simulink model "sim_Planar6DoF"  (R2017b)
settings: Solver=FixedStepAuto  StartTime=0.0  StopTime=t_end  FixedStep=Ts  RelTol=1e-3
PreLoadFcn:
  | init_sim_Planar6DoF
StopFcn:
  | runVisualization
undefined symbols (not defined in the file): B_theta, D_JointImp, D_theta, DiscIntNeverNeededParam, dq0, dq_init, K, K_JointImp, K_theta, M_des, Nb, Omega, q0, q0_offset, ROBOT, Ts
libraries: simulink x6
(part 1 of 2)
settings Model: Creator=wu_xw  LastModifiedBy=diet_ae

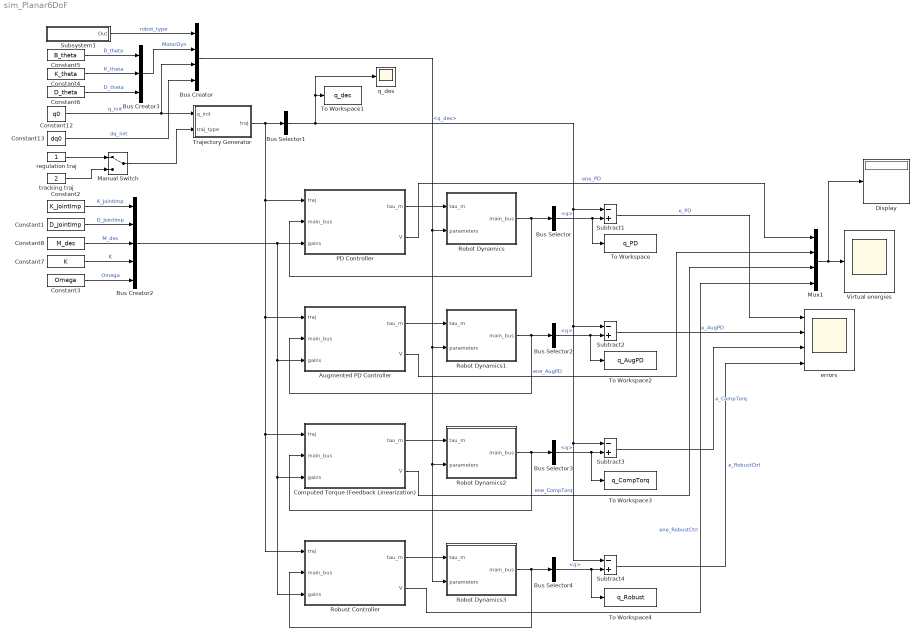
== system sim_Planar6DoF ==
  Augmented PD Controller : Subsystem
  Bus Creator : BusCreator  Inputs=4
  Bus Creator2 : BusCreator  Inputs=5
  Bus Creator3 : BusCreator  Inputs=3
  Bus Selector{,2..4} (4 alike) : BusSelector  OutputSignals=States.q
  Bus Selector1 : BusSelector  OutputSignals=q_des
  Computed Torque (Feedback Linearization) : Subsystem
  Constant1 : Constant  Value=D_JointImp  SampleTime=-1
  Constant12 : Constant  Value=q0  SampleTime=-1
  Constant13 : Constant  Value=dq0  SampleTime=-1
  Constant2 : Constant  Value=K_JointImp  SampleTime=-1
  Constant3 : Constant  Value=Omega  SampleTime=-1
  Constant4 : Constant  Value=K_theta
  Constant5 : Constant  Value=B_theta
  Constant6 : Constant  Value=D_theta
  Constant7 : Constant  Value=K  SampleTime=-1
  Constant8 : Constant  Value=M_des  SampleTime=-1
  Display : Display
  Manual Switch : ManualSwitch
  Mux1 : Mux
  PD Controller : Subsystem
  Robot Dynamics : Subsystem
      settings: MinAlgLoopOccurrences=on
      mask Display: image('Planar6DoF.png');
  Robot Dynamics1 : Subsystem
      settings: MinAlgLoopOccurrences=on
      mask Display: image('Planar6DoF.png');
  Robot Dynamics2 : Subsystem
      settings: MinAlgLoopOccurrences=on
      mask Display: image('Planar6DoF.png');
  Robot Dynamics3 : Subsystem
      settings: MinAlgLoopOccurrences=on
      mask Display: image('Planar6DoF.png');
  Robust Controller : Subsystem
  Subsystem1 : Subsystem  mask{select=1. Rigid Robot}
      mask prompts: select "Parameters are specified in"
      mask init:
      | mytab={'1. Rigid Robot',...
      |        '2. Flexible Joint Robot'};
      mask TypeOptions select: 1. Rigid Robot | 2. Flexible Joint Robot
      mask Display: disp(mytab{select});
  Subtract{1..4} (4 alike) : Sum  Inputs=-+
  To Workspace : ToWorkspace  VariableName=q_PD  SampleTime=-1
      settings: Save2DSignal=2-D array (concatenate along first dimension)
  To Workspace1 : ToWorkspace  VariableName=q_des  SampleTime=-1
      settings: Save2DSignal=2-D array (concatenate along first dimension)
  To Workspace2 : ToWorkspace  VariableName=q_AugPD  SampleTime=-1
      settings: Save2DSignal=2-D array (concatenate along first dimension)
  To Workspace3 : ToWorkspace  VariableName=q_CompTorq  SampleTime=-1
      settings: Save2DSignal=2-D array (concatenate along first dimension)
  To Workspace4 : ToWorkspace  VariableName=q_Robust  SampleTime=-1
      settings: Save2DSignal=2-D array (concatenate along first dimension)
  Trajectory Generator : Subsystem
  Virtual energies : Scope
  errors : Scope  NumInputPorts=4
  q_des : Scope
  regulation traj : Constant
  tracking traj : Constant  Value=2
  wires:
  Robot Dynamics/1(main_bus) -> Bus Selector/1, PD Controller/2(main_bus)
  PD Controller/1(tau_m) -> Robot Dynamics/1(tau_m)
  Bus Selector/1 -> Subtract1/2, To Workspace/1  "<q>"
  Constant6/1 -> Bus Creator3/3  "D_theta"
  Constant5/1 -> Bus Creator3/1  "B_theta"
  Bus Creator3/1 -> Bus Creator/2  "MotorDyn"
  Constant4/1 -> Bus Creator3/2  "K_theta"
  Constant13/1 -> Bus Creator/4  "dq_init"
  Constant12/1 -> Trajectory Generator/1(q_init), Bus Creator/3  "q_init"
  Subsystem1/1(Out) -> Bus Creator/1  "robot_type"
  Constant1/1 -> Bus Creator2/2  "D_JointImp"
  Constant2/1 -> Bus Creator2/1  "K_JointImp"
  Augmented PD Controller/1(tau_m) -> Robot Dynamics1/1(tau_m)
  Robot Dynamics2/1(main_bus) -> Bus Selector3/1, Computed Torque (Feedback Linearization)/2(main_bus)
  Computed Torque (Feedback Linearization)/1(tau_m) -> Robot Dynamics2/1(tau_m)
  Bus Selector2/1 -> To Workspace2/1, Subtract2/2  "<q>"
  Robot Dynamics1/1(main_bus) -> Augmented PD Controller/2(main_bus), Bus Selector2/1
  Bus Selector3/1 -> To Workspace3/1, Subtract3/2  "<q>"
  regulation traj/1 -> Manual Switch/1
  tracking traj/1 -> Manual Switch/2
  Manual Switch/1 -> Trajectory Generator/2(traj_type)
  Subtract1/1 -> errors/1  "e_PD"
  Subtract2/1 -> errors/2  "e_AugPD"
  Subtract3/1 -> errors/3  "e_CompTorq"
  Subtract4/1 -> errors/4  "e_RobustCtrl"
  Bus Selector1/1 -> q_des/1, To Workspace1/1, Subtract4/1, Subtract3/1, Subtract2/1, Subtract1/1  "<q_des>"
  Bus Selector4/1 -> To Workspace4/1, Subtract4/2  "<q>"
  Bus Creator/1 -> Robot Dynamics/2(parameters), Robot Dynamics3/2(parameters), Robot Dynamics2/2(parameters), Robot Dynamics1/2(parameters)
  Trajectory Generator/1(traj) -> Robust Controller/1(traj), Computed Torque (Feedback Linearization)/1(traj), Augmented PD Controller/1(traj), PD Controller/1(traj), Bus Selector1/1
  Robust Controller/1(tau_m) -> Robot Dynamics3/1(tau_m)
  Robot Dynamics3/1(main_bus) -> Robust Controller/2(main_bus), Bus Selector4/1
  Bus Creator2/1 -> Augmented PD Controller/3(gains), Robust Controller/3(gains), Computed Torque (Feedback Linearization)/3(gains), PD Controller/3(gains)
  Constant7/1 -> Bus Creator2/4  "K"
  Constant3/1 -> Bus Creator2/5  "Omega"
  Constant8/1 -> Bus Creator2/3  "M_des"
  PD Controller/2(V) -> Mux1/1  "ene_PD"
  Augmented PD Controller/2(V) -> Mux1/2  "ene_AugPD"
  Computed Torque (Feedback Linearization)/2(V) -> Mux1/3  "ene_CompTorq"
  Robust Controller/2(V) -> Mux1/4  "ene_RobustCtrl"
  Mux1/1 -> Display/1, Virtual energies/1

== system sim_Planar6DoF/Augmented PD Controller ==
  traj : Inport
  main_bus : Inport  Port=2
  gains : Inport  Port=3
  Bus Selector : BusSelector  OutputSignals=Dyn.M,Dyn.CC,Dyn.g,States.q,States.dq
  Bus Selector1 : BusSelector  OutputSignals=K_JointImp,D_JointImp
  Bus Selector2 : BusSelector  OutputSignals=q_des,dq_des,ddq_des
  Product{1..4} (4 alike) : Product  Multiplication=Matrix(*)  RndMeth=Zero
  Storage Function : Subsystem  TreatAsAtomicUnit=on
      settings: RTWFcnNameOpts=Use subsystem name  RTWFileNameOpts=Use function name
  Subtract : Sum  Inputs=+-
  Subtract1 : Sum  Inputs=--
  Subtract2 : Sum  Inputs=++++
  Subtract3 : Sum  Inputs=+-
  tau_m : Outport
  V : Outport  Port=2
  wires:
  Product4/1 -> Subtract2/2
  Bus Selector/2 -> Product4/1  "<CC>"
  Bus Selector/1 -> Storage Function/1(M), Product3/1  "<M>"
  Bus Selector2/3 -> Product3/2  "<ddq_des>"
  Subtract3/1 -> Product2/2, Storage Function/4(de)
  Bus Selector2/2 -> Subtract3/2, Product4/2  "<dq_des>"
  Bus Selector/5 -> Subtract3/1  "<dq>"
  Bus Selector2/1 -> Subtract/2  "<q_des>"
  Bus Selector/3 -> Subtract2/3  "<g>"
  Product3/1 -> Subtract2/1
  Product2/1 -> Subtract1/2
  Product1/1 -> Subtract1/1
  Bus Selector1/2 -> Product2/1  "<D_JointImp>"
  Bus Selector1/1 -> Storage Function/2(K), Product1/1  "<K_JointImp>"
  Subtract/1 -> Storage Function/3(e), Product1/2
  traj/1 -> Bus Selector2/1
  Bus Selector/4 -> Subtract/1  "<q>"
  gains/1 -> Bus Selector1/1
  main_bus/1 -> Bus Selector/1
  Subtract2/1 -> tau_m/1
  Subtract1/1 -> Subtract2/4
  Storage Function/1(V) -> V/1

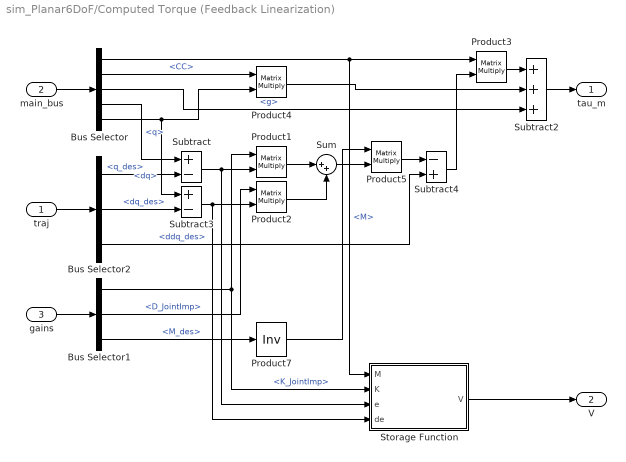
== system sim_Planar6DoF/Computed Torque (Feedback Linearization) ==
  traj : Inport
  main_bus : Inport  Port=2
  gains : Inport  Port=3
  Bus Selector : BusSelector  OutputSignals=Dyn.M,Dyn.CC,Dyn.g,States.q,States.dq
  Bus Selector1 : BusSelector  OutputSignals=K_JointImp,D_JointImp,M_des
  Bus Selector2 : BusSelector  OutputSignals=q_des,dq_des,ddq_des
  Product{1..5} (5 alike) : Product  Multiplication=Matrix(*)  RndMeth=Zero
  Product7 : Product  Inputs=/  Multiplication=Matrix(*)  RndMeth=Zero
  Storage Function : Subsystem  TreatAsAtomicUnit=on
      settings: RTWFcnNameOpts=Use subsystem name  RTWFileNameOpts=Use function name
  Subtract : Sum  Inputs=+-
  Subtract2 : Sum  Inputs=+++
  Subtract3 : Sum  Inputs=+-
  Subtract4 : Sum  Inputs=-+
  Sum : Sum  Inputs=|++
  tau_m : Outport
  V : Outport  Port=2
  wires:
  main_bus/1 -> Bus Selector/1
  Subtract2/1 -> tau_m/1
  gains/1 -> Bus Selector1/1
  Bus Selector/4 -> Subtract/1  "<q>"
  traj/1 -> Bus Selector2/1
  Subtract/1 -> Storage Function/3(e), Product1/2
  Bus Selector1/1 -> Storage Function/2(K), Product1/1  "<K_JointImp>"
  Bus Selector1/2 -> Product2/1  "<D_JointImp>"
  Product1/1 -> Sum/1
  Product2/1 -> Sum/2
  Product3/1 -> Subtract2/1
  Bus Selector/3 -> Subtract2/3  "<g>"
  Bus Selector2/1 -> Subtract/2  "<q_des>"
  Bus Selector/5 -> Product4/2, Subtract3/1  "<dq>"
  Bus Selector2/2 -> Subtract3/2  "<dq_des>"
  Subtract3/1 -> Storage Function/4(de), Product2/2
  Bus Selector2/3 -> Subtract4/2  "<ddq_des>"
  Subtract4/1 -> Product3/2
  Bus Selector/1 -> Storage Function/1(M), Product3/1  "<M>"
  Bus Selector/2 -> Product4/1  "<CC>"
  Product4/1 -> Subtract2/2
  Bus Selector1/3 -> Product7/1  "<M_des>"
  Sum/1 -> Product5/2
  Product5/1 -> Subtract4/1
  Product7/1 -> Product5/1
  Storage Function/1(V) -> V/1

== system sim_Planar6DoF/PD Controller ==
  traj : Inport
  main_bus : Inport  Port=2
  gains : Inport  Port=3
  Bus Selector : BusSelector  OutputSignals=Dyn.g,States.q,States.dq,Dyn.M
  Bus Selector1 : BusSelector  OutputSignals=K_JointImp,D_JointImp
  Bus Selector2 : BusSelector  OutputSignals=q_des,dq_des
  Gain : Gain  Gain=-1
  Product1 : Product  Multiplication=Matrix(*)  RndMeth=Zero
  Product2 : Product  Multiplication=Matrix(*)  RndMeth=Zero
  Storage Function : Subsystem  TreatAsAtomicUnit=on
      settings: RTWFcnNameOpts=Use subsystem name  RTWFileNameOpts=Use function name
  Subtract : Sum  Inputs=+-
  Subtract1 : Sum
  Subtract2 : Sum
  Subtract3 : Sum  Inputs=+-
  tau_m : Outport
  V : Outport  Port=2
  wires:
  main_bus/1 -> Bus Selector/1
  Bus Selector/3 -> Subtract3/1, Product2/2  "<dq>"
  Subtract2/1 -> tau_m/1
  gains/1 -> Bus Selector1/1
  Bus Selector/2 -> Subtract/1  "<q>"
  traj/1 -> Bus Selector2/1
  Subtract/1 -> Storage Function/3(e), Product1/2
  Bus Selector1/1 -> Storage Function/2(K), Product1/1  "<K_JointImp>"
  Bus Selector1/2 -> Product2/1  "<D_JointImp>"
  Product1/1 -> Subtract1/1
  Product2/1 -> Subtract1/2
  Subtract1/1 -> Gain/1
  Gain/1 -> Subtract2/2
  Bus Selector/1 -> Subtract2/1  "<g>"
  Bus Selector2/1 -> Subtract/2  "<q_des>"
  Bus Selector/4 -> Storage Function/1(M)  "<M>"
  Subtract3/1 -> Storage Function/4(de)
  Bus Selector2/2 -> Subtract3/2  "<dq_des>"
  Storage Function/1(V) -> V/1

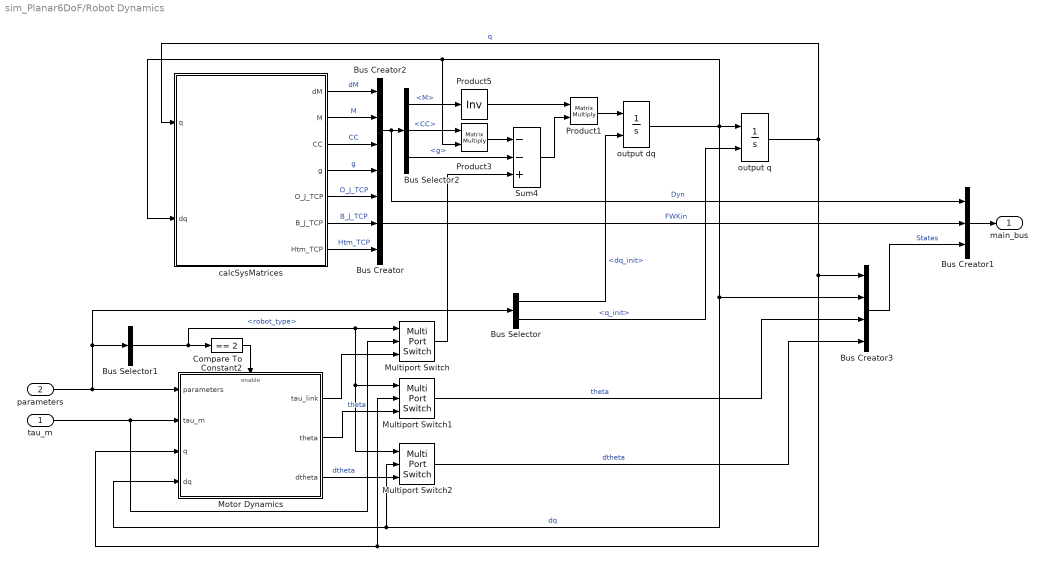
== system sim_Planar6DoF/Robot Dynamics ==
  tau_m : Inport
  parameters : Inport  Port=2
  Bus Creator : BusCreator  Inputs=3
  Bus Creator1 : BusCreator  Inputs=3
  Bus Creator2 : BusCreator  Inputs=4
  Bus Creator3 : BusCreator  Inputs=4
  Bus Selector : BusSelector  OutputSignals=dq_init,q_init
  Bus Selector1 : BusSelector  OutputSignals=robot_type
  Bus Selector2 : BusSelector  OutputSignals=M,CC,g
  Compare To Constant2 : simulink/Logic and Bit Operations/Compare To Constant  relop===  const=2  OutDataTypeStr=boolean
  Motor Dynamics : Subsystem  TreatAsAtomicUnit=on
  Multiport Switch : MultiPortSwitch  Inputs=2
  Multiport Switch1 : MultiPortSwitch  Inputs=2
  Multiport Switch2 : MultiPortSwitch  Inputs=2
  Product1 : Product  Multiplication=Matrix(*)  RndMeth=Zero
  Product3 : Product  Multiplication=Matrix(*)  RndMeth=Zero
  Product5 : Product  Inputs=/  Multiplication=Matrix(*)  RndMeth=Zero
  Sum4 : Sum  Inputs=--+
  calcSysMatrices : MATLAB Function  TreatAsAtomicUnit=on  mask{ROBOT=ROBOT}
      mask prompts: ROBOT "Robot Model"
      mask help:
      | Calculates inertia and coriolis compensation matrices
      |
      | A MATLAB structure ROBOT with the fields:
      |
      | g0 - matrix stacking vertically the homogeneous transformation matrices from parent to link in the zero-configuration
      | csi - vector stacking vertically the 6-by-1 relative body jacobian (twist) in link frame
      | Mass - block diagonal matrix, where each block is the 6-by-6 inertia matrix of the link in link frame
      |
      | must be initialized in workspace.
  output dq : Integrator  InitialConditionSource=external  InitialCondition=[zeros(Nb,1); dq_init]
  output q : Integrator  InitialConditionSource=external  InitialCondition=[zeros(Nb,1); dq_init]
  main_bus : Outport
  wires:
  Sum4/1 -> Product1/2
  parameters/1 -> Bus Selector/1, Bus Selector1/1, Motor Dynamics/1(parameters)
  Bus Selector/1 -> output dq/2  "<dq_init>"
  Product1/1 -> output dq/1
  Bus Creator1/1 -> main_bus/1
  Product3/1 -> Sum4/1
  Bus Selector/2 -> output q/2  "<q_init>"
  calcSysMatrices/2(M) -> Bus Creator2/2  "M"
  Product5/1 -> Product1/1
  calcSysMatrices/3(CC) -> Bus Creator2/3  "CC"
  output dq/1 -> output q/1, calcSysMatrices/2(dq), Product3/2, Bus Creator3/2, Multiport Switch2/2, Motor Dynamics/4(dq)  "dq"
  calcSysMatrices/4(g) -> Bus Creator2/4  "g"
  calcSysMatrices/5(O_J_TCP) -> Bus Creator/1  "O_J_TCP"
  calcSysMatrices/6(B_J_TCP) -> Bus Creator/2  "B_J_TCP"
  calcSysMatrices/7(Htm_TCP) -> Bus Creator/3  "Htm_TCP"
  Bus Creator/1 -> Bus Creator1/2  "FWKin"
  Bus Selector1/1 -> Multiport Switch2/1, Multiport Switch1/1, Multiport Switch/1, Compare To Constant2/1  "<robot_type>"
  Compare To Constant2/1 -> Motor Dynamics/Enable
  tau_m/1 -> Multiport Switch/2, Motor Dynamics/2(tau_m)
  Motor Dynamics/1(tau_link) -> Multiport Switch/3
  Multiport Switch1/1 -> Bus Creator3/3  "theta"
  Multiport Switch2/1 -> Bus Creator3/4  "dtheta"
  Multiport Switch/1 -> Sum4/3
  Motor Dynamics/2(theta) -> Multiport Switch1/3  "theta"
  Motor Dynamics/3(dtheta) -> Multiport Switch2/3  "dtheta"
  Bus Creator3/1 -> Bus Creator1/3  "States"
  calcSysMatrices/1(dM) -> Bus Creator2/1  "dM"
  Bus Creator2/1 -> Bus Creator1/1, Bus Selector2/1  "Dyn"
  Bus Selector2/1 -> Product5/1  "<M>"
  Bus Selector2/2 -> Product3/1  "<CC>"
  Bus Selector2/3 -> Sum4/2  "<g>"
  output q/1 -> calcSysMatrices/1(q), Bus Creator3/1, Multiport Switch1/2, Motor Dynamics/3(q)  "q"

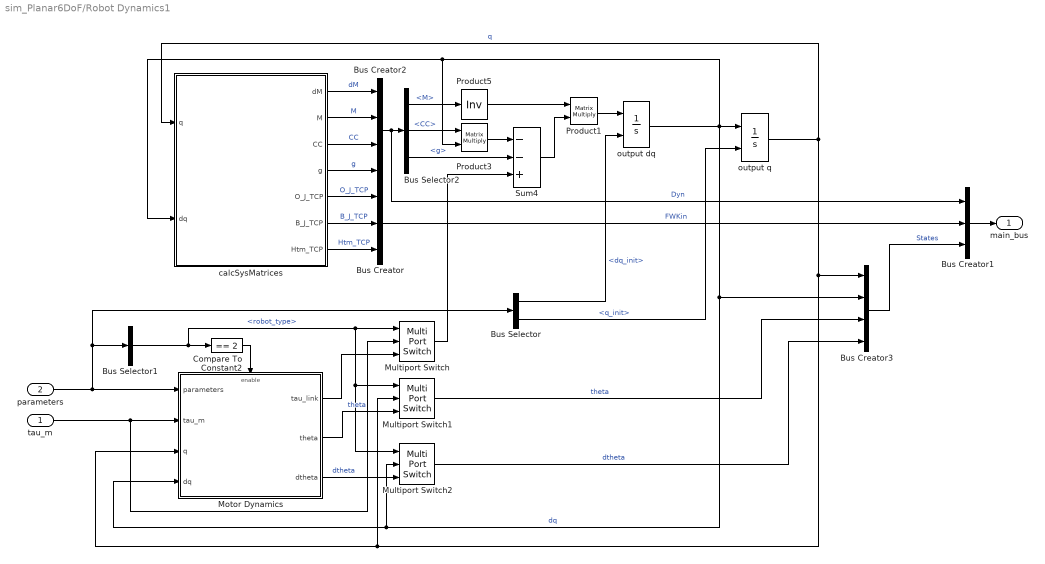
== system sim_Planar6DoF/Robot Dynamics1 ==
  tau_m : Inport
  parameters : Inport  Port=2
  Bus Creator : BusCreator  Inputs=3
  Bus Creator1 : BusCreator  Inputs=3
  Bus Creator2 : BusCreator  Inputs=4
  Bus Creator3 : BusCreator  Inputs=4
  Bus Selector : BusSelector  OutputSignals=dq_init,q_init
  Bus Selector1 : BusSelector  OutputSignals=robot_type
  Bus Selector2 : BusSelector  OutputSignals=M,CC,g
  Compare To Constant2 : simulink/Logic and Bit Operations/Compare To Constant  relop===  const=2  OutDataTypeStr=boolean
  Motor Dynamics : Subsystem  TreatAsAtomicUnit=on
  Multiport Switch : MultiPortSwitch  Inputs=2
  Multiport Switch1 : MultiPortSwitch  Inputs=2
  Multiport Switch2 : MultiPortSwitch  Inputs=2
  Product1 : Product  Multiplication=Matrix(*)  RndMeth=Zero
  Product3 : Product  Multiplication=Matrix(*)  RndMeth=Zero
  Product5 : Product  Inputs=/  Multiplication=Matrix(*)  RndMeth=Zero
  Sum4 : Sum  Inputs=--+
  calcSysMatrices : MATLAB Function  TreatAsAtomicUnit=on  mask{ROBOT=ROBOT}
      mask prompts: ROBOT "Robot Model"
      mask help:
      | Calculates inertia and coriolis compensation matrices
      |
      | A MATLAB structure ROBOT with the fields:
      |
      | g0 - matrix stacking vertically the homogeneous transformation matrices from parent to link in the zero-configuration
      | csi - vector stacking vertically the 6-by-1 relative body jacobian (twist) in link frame
      | Mass - block diagonal matrix, where each block is the 6-by-6 inertia matrix of the link in link frame
      |
      | must be initialized in workspace.
  output dq : Integrator  InitialConditionSource=external  InitialCondition=[zeros(Nb,1); dq_init]
  output q : Integrator  InitialConditionSource=external  InitialCondition=[zeros(Nb,1); dq_init]
  main_bus : Outport
  wires:
  output q/1 -> Motor Dynamics/3(q), Multiport Switch1/2, Bus Creator3/1, calcSysMatrices/1(q)  "q"
  Bus Selector2/3 -> Sum4/2  "<g>"
  Bus Selector2/2 -> Product3/1  "<CC>"
  Bus Selector2/1 -> Product5/1  "<M>"
  Bus Creator2/1 -> Bus Selector2/1, Bus Creator1/1  "Dyn"
  calcSysMatrices/1(dM) -> Bus Creator2/1  "dM"
  Bus Creator3/1 -> Bus Creator1/3  "States"
  Motor Dynamics/3(dtheta) -> Multiport Switch2/3  "dtheta"
  Motor Dynamics/2(theta) -> Multiport Switch1/3  "theta"
  Multiport Switch/1 -> Sum4/3
  Multiport Switch2/1 -> Bus Creator3/4  "dtheta"
  Multiport Switch1/1 -> Bus Creator3/3  "theta"
  Motor Dynamics/1(tau_link) -> Multiport Switch/3
  tau_m/1 -> Motor Dynamics/2(tau_m), Multiport Switch/2
  Compare To Constant2/1 -> Motor Dynamics/Enable
  Bus Selector1/1 -> Compare To Constant2/1, Multiport Switch/1, Multiport Switch1/1, Multiport Switch2/1  "<robot_type>"
  Bus Creator/1 -> Bus Creator1/2  "FWKin"
  calcSysMatrices/7(Htm_TCP) -> Bus Creator/3  "Htm_TCP"
  calcSysMatrices/6(B_J_TCP) -> Bus Creator/2  "B_J_TCP"
  calcSysMatrices/5(O_J_TCP) -> Bus Creator/1  "O_J_TCP"
  calcSysMatrices/4(g) -> Bus Creator2/4  "g"
  output dq/1 -> Motor Dynamics/4(dq), Multiport Switch2/2, Bus Creator3/2, Product3/2, calcSysMatrices/2(dq), output q/1  "dq"
  calcSysMatrices/3(CC) -> Bus Creator2/3  "CC"
  Product5/1 -> Product1/1
  calcSysMatrices/2(M) -> Bus Creator2/2  "M"
  Bus Selector/2 -> output q/2  "<q_init>"
  Product3/1 -> Sum4/1
  Bus Creator1/1 -> main_bus/1
  Product1/1 -> output dq/1
  Bus Selector/1 -> output dq/2  "<dq_init>"
  parameters/1 -> Motor Dynamics/1(parameters), Bus Selector1/1, Bus Selector/1
  Sum4/1 -> Product1/2

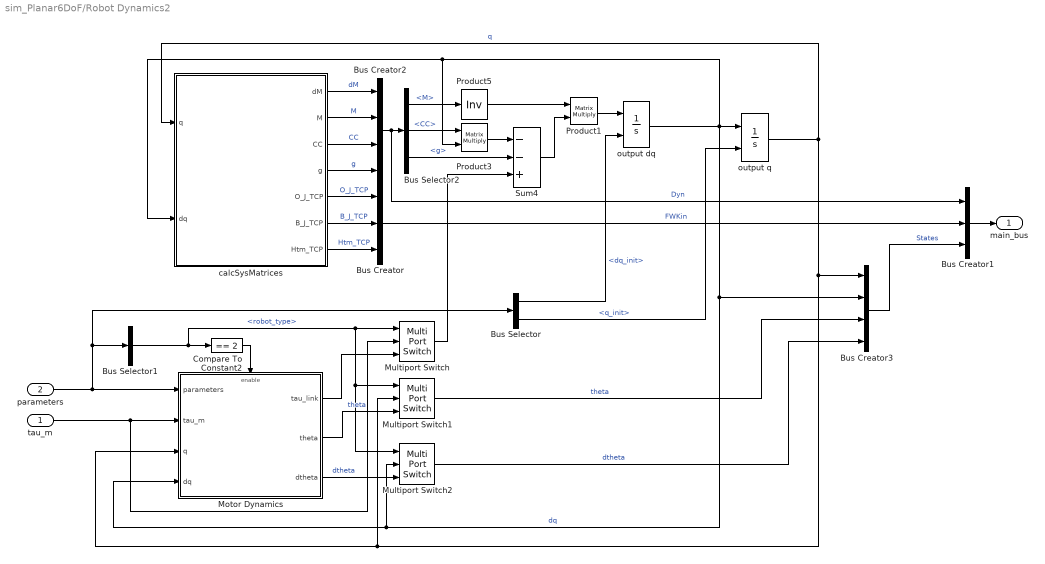
== system sim_Planar6DoF/Robot Dynamics2 ==
  tau_m : Inport
  parameters : Inport  Port=2
  Bus Creator : BusCreator  Inputs=3
  Bus Creator1 : BusCreator  Inputs=3
  Bus Creator2 : BusCreator  Inputs=4
  Bus Creator3 : BusCreator  Inputs=4
  Bus Selector : BusSelector  OutputSignals=dq_init,q_init
  Bus Selector1 : BusSelector  OutputSignals=robot_type
  Bus Selector2 : BusSelector  OutputSignals=M,CC,g
  Compare To Constant2 : simulink/Logic and Bit Operations/Compare To Constant  relop===  const=2  OutDataTypeStr=boolean
  Motor Dynamics : Subsystem  TreatAsAtomicUnit=on
  Multiport Switch : MultiPortSwitch  Inputs=2
  Multiport Switch1 : MultiPortSwitch  Inputs=2
  Multiport Switch2 : MultiPortSwitch  Inputs=2
  Product1 : Product  Multiplication=Matrix(*)  RndMeth=Zero
  Product3 : Product  Multiplication=Matrix(*)  RndMeth=Zero
  Product5 : Product  Inputs=/  Multiplication=Matrix(*)  RndMeth=Zero
  Sum4 : Sum  Inputs=--+
  calcSysMatrices : MATLAB Function  TreatAsAtomicUnit=on  mask{ROBOT=ROBOT}
      mask prompts: ROBOT "Robot Model"
      mask help:
      | Calculates inertia and coriolis compensation matrices
      |
      | A MATLAB structure ROBOT with the fields:
      |
      | g0 - matrix stacking vertically the homogeneous transformation matrices from parent to link in the zero-configuration
      | csi - vector stacking vertically the 6-by-1 relative body jacobian (twist) in link frame
      | Mass - block diagonal matrix, where each block is the 6-by-6 inertia matrix of the link in link frame
      |
      | must be initialized in workspace.
  output dq : Integrator  InitialConditionSource=external  InitialCondition=[zeros(Nb,1); dq_init]
  output q : Integrator  InitialConditionSource=external  InitialCondition=[zeros(Nb,1); dq_init]
  main_bus : Outport
  wires:
  Sum4/1 -> Product1/2
  parameters/1 -> Bus Selector/1, Bus Selector1/1, Motor Dynamics/1(parameters)
  Bus Selector/1 -> output dq/2  "<dq_init>"
  Product1/1 -> output dq/1
  Bus Creator1/1 -> main_bus/1
  Product3/1 -> Sum4/1
  Bus Selector/2 -> output q/2  "<q_init>"
  calcSysMatrices/2(M) -> Bus Creator2/2  "M"
  Product5/1 -> Product1/1
  calcSysMatrices/3(CC) -> Bus Creator2/3  "CC"
  output dq/1 -> output q/1, calcSysMatrices/2(dq), Product3/2, Bus Creator3/2, Multiport Switch2/2, Motor Dynamics/4(dq)  "dq"
  calcSysMatrices/4(g) -> Bus Creator2/4  "g"
  calcSysMatrices/5(O_J_TCP) -> Bus Creator/1  "O_J_TCP"
  calcSysMatrices/6(B_J_TCP) -> Bus Creator/2  "B_J_TCP"
  calcSysMatrices/7(Htm_TCP) -> Bus Creator/3  "Htm_TCP"
  Bus Creator/1 -> Bus Creator1/2  "FWKin"
  Bus Selector1/1 -> Multiport Switch2/1, Multiport Switch1/1, Multiport Switch/1, Compare To Constant2/1  "<robot_type>"
  Compare To Constant2/1 -> Motor Dynamics/Enable
  tau_m/1 -> Multiport Switch/2, Motor Dynamics/2(tau_m)
  Motor Dynamics/1(tau_link) -> Multiport Switch/3
  Multiport Switch1/1 -> Bus Creator3/3  "theta"
  Multiport Switch2/1 -> Bus Creator3/4  "dtheta"
  Multiport Switch/1 -> Sum4/3
  Motor Dynamics/2(theta) -> Multiport Switch1/3  "theta"
  Motor Dynamics/3(dtheta) -> Multiport Switch2/3  "dtheta"
  Bus Creator3/1 -> Bus Creator1/3  "States"
  calcSysMatrices/1(dM) -> Bus Creator2/1  "dM"
  Bus Creator2/1 -> Bus Creator1/1, Bus Selector2/1  "Dyn"
  Bus Selector2/1 -> Product5/1  "<M>"
  Bus Selector2/2 -> Product3/1  "<CC>"
  Bus Selector2/3 -> Sum4/2  "<g>"
  output q/1 -> calcSysMatrices/1(q), Bus Creator3/1, Multiport Switch1/2, Motor Dynamics/3(q)  "q"

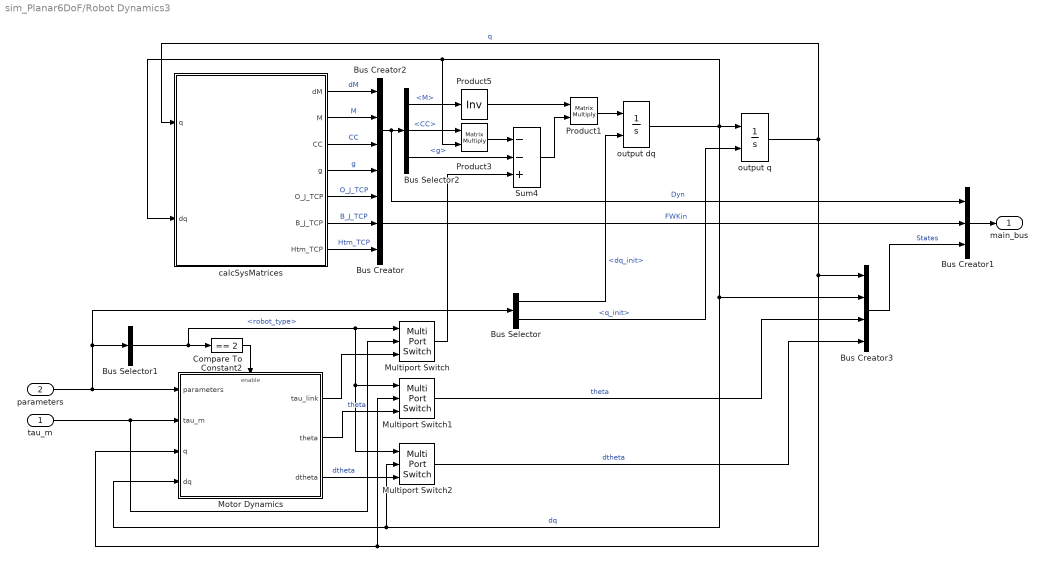
== system sim_Planar6DoF/Robot Dynamics3 ==
  tau_m : Inport
  parameters : Inport  Port=2
  Bus Creator : BusCreator  Inputs=3
  Bus Creator1 : BusCreator  Inputs=3
  Bus Creator2 : BusCreator  Inputs=4
  Bus Creator3 : BusCreator  Inputs=4
  Bus Selector : BusSelector  OutputSignals=dq_init,q_init
  Bus Selector1 : BusSelector  OutputSignals=robot_type
  Bus Selector2 : BusSelector  OutputSignals=M,CC,g
  Compare To Constant2 : simulink/Logic and Bit Operations/Compare To Constant  relop===  const=2  OutDataTypeStr=boolean
  Motor Dynamics : Subsystem  TreatAsAtomicUnit=on
  Multiport Switch : MultiPortSwitch  Inputs=2
  Multiport Switch1 : MultiPortSwitch  Inputs=2
  Multiport Switch2 : MultiPortSwitch  Inputs=2
  Product1 : Product  Multiplication=Matrix(*)  RndMeth=Zero
  Product3 : Product  Multiplication=Matrix(*)  RndMeth=Zero
  Product5 : Product  Inputs=/  Multiplication=Matrix(*)  RndMeth=Zero
  Sum4 : Sum  Inputs=--+
  calcSysMatrices : MATLAB Function  TreatAsAtomicUnit=on  mask{ROBOT=ROBOT}
      mask prompts: ROBOT "Robot Model"
      mask help:
      | Calculates inertia and coriolis compensation matrices
      |
      | A MATLAB structure ROBOT with the fields:
      |
      | g0 - matrix stacking vertically the homogeneous transformation matrices from parent to link in the zero-configuration
      | csi - vector stacking vertically the 6-by-1 relative body jacobian (twist) in link frame
      | Mass - block diagonal matrix, where each block is the 6-by-6 inertia matrix of the link in link frame
      |
      | must be initialized in workspace.
  output dq : Integrator  InitialConditionSource=external  InitialCondition=[zeros(Nb,1); dq_init]
  output q : Integrator  InitialConditionSource=external  InitialCondition=[zeros(Nb,1); dq_init]
  main_bus : Outport
  wires:
  output q/1 -> Motor Dynamics/3(q), Multiport Switch1/2, Bus Creator3/1, calcSysMatrices/1(q)  "q"
  Bus Selector2/3 -> Sum4/2  "<g>"
  Bus Selector2/2 -> Product3/1  "<CC>"
  Bus Selector2/1 -> Product5/1  "<M>"
  Bus Creator2/1 -> Bus Selector2/1, Bus Creator1/1  "Dyn"
  calcSysMatrices/1(dM) -> Bus Creator2/1  "dM"
  Bus Creator3/1 -> Bus Creator1/3  "States"
  Motor Dynamics/3(dtheta) -> Multiport Switch2/3  "dtheta"
  Motor Dynamics/2(theta) -> Multiport Switch1/3  "theta"
  Multiport Switch/1 -> Sum4/3
  Multiport Switch2/1 -> Bus Creator3/4  "dtheta"
  Multiport Switch1/1 -> Bus Creator3/3  "theta"
  Motor Dynamics/1(tau_link) -> Multiport Switch/3
  tau_m/1 -> Motor Dynamics/2(tau_m), Multiport Switch/2
  Compare To Constant2/1 -> Motor Dynamics/Enable
  Bus Selector1/1 -> Compare To Constant2/1, Multiport Switch/1, Multiport Switch1/1, Multiport Switch2/1  "<robot_type>"
  Bus Creator/1 -> Bus Creator1/2  "FWKin"
  calcSysMatrices/7(Htm_TCP) -> Bus Creator/3  "Htm_TCP"
  calcSysMatrices/6(B_J_TCP) -> Bus Creator/2  "B_J_TCP"
  calcSysMatrices/5(O_J_TCP) -> Bus Creator/1  "O_J_TCP"
  calcSysMatrices/4(g) -> Bus Creator2/4  "g"
  output dq/1 -> Motor Dynamics/4(dq), Multiport Switch2/2, Bus Creator3/2, Product3/2, calcSysMatrices/2(dq), output q/1  "dq"
  calcSysMatrices/3(CC) -> Bus Creator2/3  "CC"
  Product5/1 -> Product1/1
  calcSysMatrices/2(M) -> Bus Creator2/2  "M"
  Bus Selector/2 -> output q/2  "<q_init>"
  Product3/1 -> Sum4/1
  Bus Creator1/1 -> main_bus/1
  Product1/1 -> output dq/1
  Bus Selector/1 -> output dq/2  "<dq_init>"
  parameters/1 -> Motor Dynamics/1(parameters), Bus Selector1/1, Bus Selector/1
  Sum4/1 -> Product1/2

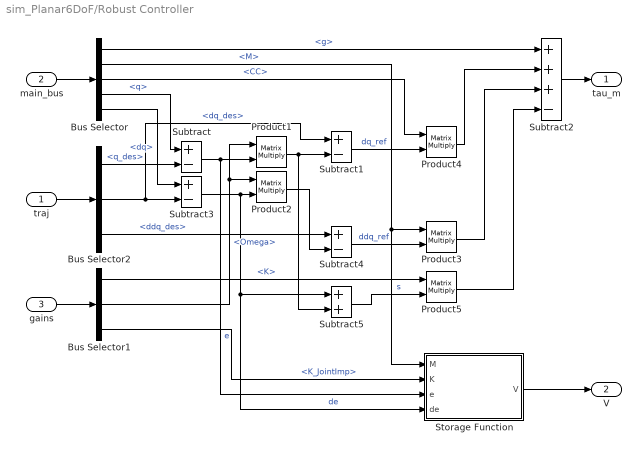
== system sim_Planar6DoF/Robust Controller ==
  traj : Inport
  main_bus : Inport  Port=2
  gains : Inport  Port=3
  Bus Selector : BusSelector  OutputSignals=Dyn.g,Dyn.M,Dyn.CC,States.q,States.dq
  Bus Selector1 : BusSelector  OutputSignals=K,Omega,K_JointImp
  Bus Selector2 : BusSelector  OutputSignals=q_des,dq_des,ddq_des
  Product{1..5} (5 alike) : Product  Multiplication=Matrix(*)  RndMeth=Zero
  Storage Function : Subsystem  TreatAsAtomicUnit=on
      settings: RTWFcnNameOpts=Use subsystem name  RTWFileNameOpts=Use function name
  Subtract{,1,3..4} (4 alike) : Sum  Inputs=+-
  Subtract2 : Sum  Inputs=+++-
  Subtract5 : Sum
  tau_m : Outport
  V : Outport  Port=2
  wires:
  Bus Selector/3 -> Product4/1  "<CC>"
  Bus Selector/2 -> Storage Function/1(M), Product3/1  "<M>"
  Bus Selector2/3 -> Subtract4/1  "<ddq_des>"
  Subtract3/1 -> Product2/2, Storage Function/4(de), Subtract5/1  "de"
  Bus Selector2/2 -> Subtract1/1, Subtract3/2  "<dq_des>"
  Bus Selector/5 -> Subtract3/1  "<dq>"
  Bus Selector2/1 -> Subtract/2  "<q_des>"
  Bus Selector/1 -> Subtract2/1  "<g>"
  Product3/1 -> Subtract2/3
  Product2/1 -> Subtract4/2
  Product1/1 -> Subtract5/2, Subtract1/2
  Subtract/1 -> Storage Function/3(e), Product1/2  "e"
  traj/1 -> Bus Selector2/1
  Bus Selector/4 -> Subtract/1  "<q>"
  gains/1 -> Bus Selector1/1
  Subtract2/1 -> tau_m/1
  main_bus/1 -> Bus Selector/1
  Bus Selector1/2 -> Product2/1, Product1/1  "<Omega>"
  Subtract1/1 -> Product4/2  "dq_ref"
  Subtract4/1 -> Product3/2  "ddq_ref"
  Product5/1 -> Subtract2/4
  Bus Selector1/1 -> Product5/1  "<K>"
  Subtract5/1 -> Product5/2  "s"
  Product4/1 -> Subtract2/2
  Storage Function/1(V) -> V/1
  Bus Selector1/3 -> Storage Function/2(K)  "<K_JointImp>"

== system sim_Planar6DoF/Subsystem1 ==
  Constant : Constant  Value=select  SampleTime=-1
  Out : Outport
  wires:
  Constant/1 -> Out/1

== system sim_Planar6DoF/Trajectory Generator ==
  q_init : Inport
  traj_type : Inport  Port=2
  Bus Creator1 : BusCreator  Inputs=3
  Bus Creator2 : BusCreator  Inputs=3
  Compare To Constant2 : simulink/Logic and Bit Operations/Compare To Constant  relop===  const=2  OutDataTypeStr=boolean
  Compare To Constant3 : simulink/Logic and Bit Operations/Compare To Constant  relop===  const=1  OutDataTypeStr=boolean
  Multiport Switch4 : MultiPortSwitch  Inputs=2
  Regulation Traj : Subsystem
  Sum1 : Sum  Inputs=++|
  Sum2 : Sum  Inputs=++|
  Tracking Traj : Subsystem
  traj : Outport
  wires:
  Sum2/1 -> Bus Creator2/1  "q_des"
  Regulation Traj/2(dq_des) -> Bus Creator2/2  "dq_des"
  Bus Creator2/1 -> Multiport Switch4/2
  Regulation Traj/3(ddq_des) -> Bus Creator2/3  "ddq_des"
  Compare To Constant3/1 -> Regulation Traj/Enable
  Compare To Constant2/1 -> Tracking Traj/Enable
  traj_type/1 -> Multiport Switch4/1, Compare To Constant2/1, Compare To Constant3/1
  Tracking Traj/3(ddq_des) -> Bus Creator1/3  "ddq_des"
  Bus Creator1/1 -> Multiport Switch4/3
  Tracking Traj/1(q_dev) -> Sum1/2
  Tracking Traj/2(dq_des) -> Bus Creator1/2  "dq_des"
  Sum1/1 -> Bus Creator1/1  "q_des"
  Regulation Traj/1(q_dev) -> Sum2/2
  q_init/1 -> Sum1/1, Sum2/1
  Multiport Switch4/1 -> traj/1

== system sim_Planar6DoF/Augmented PD Controller/Storage Function ==
  M : Inport
  K : Inport  Port=2
  e : Inport  Port=3
  de : Inport  Port=4
  Add1 : Sum
  Gain : Gain  Gain=0.5
  Math Function : Math  Operator=transpose  SaturateOnIntegerOverflow=on
  Math Function1 : Math  Operator=transpose  SaturateOnIntegerOverflow=on
  Product{1..4} (4 alike) : Product  Multiplication=Matrix(*)  RndMeth=Zero
  V_kin : Scope
  V_pot : Scope
  V_total : Scope
  V : Outport
  wires:
  Product2/1 -> Gain/1
  Gain/1 -> Add1/1, V_kin/1
  Product4/1 -> Product2/1
  de/1 -> Product2/2, Math Function/1
  Math Function/1 -> Product4/1
  M/1 -> Product4/2
  K/1 -> Product3/2
  Math Function1/1 -> Product3/1
  e/1 -> Product1/2, Math Function1/1
  Product3/1 -> Product1/1
  Product1/1 -> Add1/2, V_pot/1
  Add1/1 -> V_total/1, V/1

== system sim_Planar6DoF/Computed Torque (Feedback Linearization)/Storage Function ==
  M : Inport
  K : Inport  Port=2
  e : Inport  Port=3
  de : Inport  Port=4
  Add1 : Sum
  Gain : Gain  Gain=0.5
  Math Function : Math  Operator=transpose  SaturateOnIntegerOverflow=on
  Math Function1 : Math  Operator=transpose  SaturateOnIntegerOverflow=on
  Product{1..4} (4 alike) : Product  Multiplication=Matrix(*)  RndMeth=Zero
  V_kin : Scope
  V_pot : Scope
  V_total : Scope
  V : Outport
  wires:
  Product2/1 -> Gain/1
  Gain/1 -> Add1/1, V_kin/1
  Product4/1 -> Product2/1
  de/1 -> Product2/2, Math Function/1
  Math Function/1 -> Product4/1
  M/1 -> Product4/2
  K/1 -> Product3/2
  Math Function1/1 -> Product3/1
  e/1 -> Product1/2, Math Function1/1
  Product3/1 -> Product1/1
  Product1/1 -> Add1/2, V_pot/1
  Add1/1 -> V_total/1, V/1

== system sim_Planar6DoF/PD Controller/Storage Function ==
  M : Inport
  K : Inport  Port=2
  e : Inport  Port=3
  de : Inport  Port=4
  Add1 : Sum
  Gain : Gain  Gain=0.5
  Math Function : Math  Operator=transpose  SaturateOnIntegerOverflow=on
  Math Function1 : Math  Operator=transpose  SaturateOnIntegerOverflow=on
  Product{1..4} (4 alike) : Product  Multiplication=Matrix(*)  RndMeth=Zero
  V_kin : Scope
  V_pot : Scope
  V_total : Scope
  V : Outport
  wires:
  Product2/1 -> Gain/1
  Gain/1 -> Add1/1, V_kin/1
  Product4/1 -> Product2/1
  de/1 -> Product2/2, Math Function/1
  Math Function/1 -> Product4/1
  M/1 -> Product4/2
  K/1 -> Product3/2
  Math Function1/1 -> Product3/1
  e/1 -> Product1/2, Math Function1/1
  Product3/1 -> Product1/1
  Product1/1 -> Add1/2, V_pot/1
  Add1/1 -> V_total/1, V/1

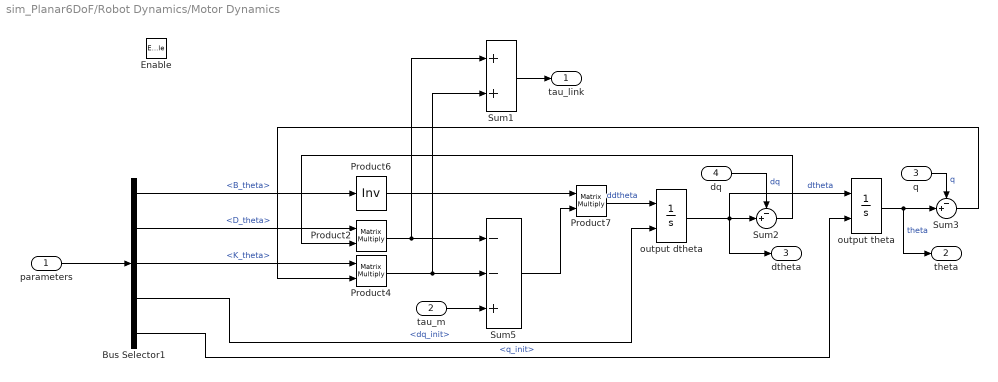
== system sim_Planar6DoF/Robot Dynamics/Motor Dynamics ==
  parameters : Inport
  tau_m : Inport  Port=2
  q : Inport  Port=3
  dq : Inport  Port=4
  Enable : EnablePort
  Bus Selector1 : BusSelector  OutputSignals=MotorDyn.B_theta,MotorDyn.D_theta,MotorDyn.K_theta,dq_init,q_init
  Product2 : Product  Multiplication=Matrix(*)  RndMeth=Zero
  Product4 : Product  Multiplication=Matrix(*)  RndMeth=Zero
  Product6 : Product  Inputs=/  Multiplication=Matrix(*)  RndMeth=Zero
  Product7 : Product  Multiplication=Matrix(*)  RndMeth=Zero
  Sum1 : Sum
  Sum2 : Sum  Inputs=-+|
  Sum3 : Sum  Inputs=-+|
  Sum5 : Sum  Inputs=--+
  output dtheta : Integrator  InitialConditionSource=external  InitialCondition=[zeros(Nb,1); dq_init]
  output theta : Integrator  InitialConditionSource=external  InitialCondition=[zeros(Nb,1); dq_init]
  tau_link : Outport
  theta : Outport  Port=2
  dtheta : Outport  Port=3
  wires:
  Bus Selector1/4 -> output dtheta/2  "<dq_init>"
  output dtheta/1 -> output theta/1, dtheta/1, Sum2/2  "dtheta"
  Product7/1 -> output dtheta/1  "ddtheta"
  Sum5/1 -> Product7/2
  Bus Selector1/1 -> Product6/1  "<B_theta>"
  Bus Selector1/3 -> Product4/1  "<K_theta>"
  tau_m/1 -> Sum5/3
  Bus Selector1/5 -> output theta/2  "<q_init>"
  Product6/1 -> Product7/1
  Sum2/1 -> Product2/2
  Bus Selector1/2 -> Product2/1  "<D_theta>"
  Product4/1 -> Sum1/2, Sum5/2
  Sum3/1 -> Product4/2
  output theta/1 -> theta/1, Sum3/2  "theta"
  dq/1 -> Sum2/1  "dq"
  q/1 -> Sum3/1  "q"
  Product2/1 -> Sum1/1, Sum5/1
  parameters/1 -> Bus Selector1/1
  Sum1/1 -> tau_link/1

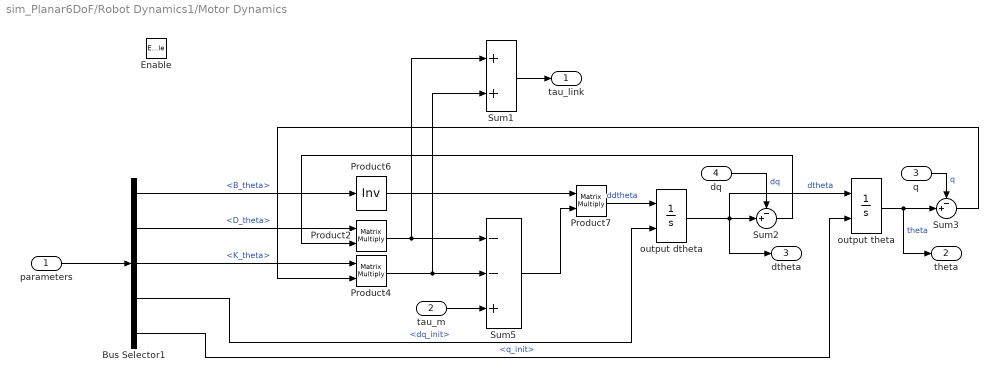
== system sim_Planar6DoF/Robot Dynamics1/Motor Dynamics ==
  parameters : Inport
  tau_m : Inport  Port=2
  q : Inport  Port=3
  dq : Inport  Port=4
  Enable : EnablePort
  Bus Selector1 : BusSelector  OutputSignals=MotorDyn.B_theta,MotorDyn.D_theta,MotorDyn.K_theta,dq_init,q_init
  Product2 : Product  Multiplication=Matrix(*)  RndMeth=Zero
  Product4 : Product  Multiplication=Matrix(*)  RndMeth=Zero
  Product6 : Product  Inputs=/  Multiplication=Matrix(*)  RndMeth=Zero
  Product7 : Product  Multiplication=Matrix(*)  RndMeth=Zero
  Sum1 : Sum
  Sum2 : Sum  Inputs=-+|
  Sum3 : Sum  Inputs=-+|
  Sum5 : Sum  Inputs=--+
  output dtheta : Integrator  InitialConditionSource=external  InitialCondition=[zeros(Nb,1); dq_init]
  output theta : Integrator  InitialConditionSource=external  InitialCondition=[zeros(Nb,1); dq_init]
  tau_link : Outport
  theta : Outport  Port=2
  dtheta : Outport  Port=3
  wires:
  Sum1/1 -> tau_link/1
  parameters/1 -> Bus Selector1/1
  Product2/1 -> Sum5/1, Sum1/1
  q/1 -> Sum3/1  "q"
  dq/1 -> Sum2/1  "dq"
  output theta/1 -> Sum3/2, theta/1  "theta"
  Sum3/1 -> Product4/2
  Product4/1 -> Sum5/2, Sum1/2
  Bus Selector1/2 -> Product2/1  "<D_theta>"
  Sum2/1 -> Product2/2
  Product6/1 -> Product7/1
  Bus Selector1/5 -> output theta/2  "<q_init>"
  tau_m/1 -> Sum5/3
  Bus Selector1/3 -> Product4/1  "<K_theta>"
  Bus Selector1/1 -> Product6/1  "<B_theta>"
  Sum5/1 -> Product7/2
  Product7/1 -> output dtheta/1  "ddtheta"
  output dtheta/1 -> Sum2/2, dtheta/1, output theta/1  "dtheta"
  Bus Selector1/4 -> output dtheta/2  "<dq_init>"

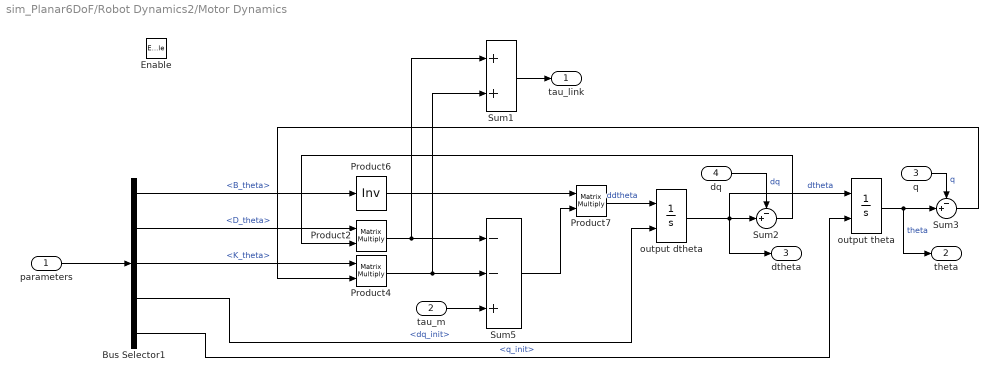
== system sim_Planar6DoF/Robot Dynamics2/Motor Dynamics ==
  parameters : Inport
  tau_m : Inport  Port=2
  q : Inport  Port=3
  dq : Inport  Port=4
  Enable : EnablePort
  Bus Selector1 : BusSelector  OutputSignals=MotorDyn.B_theta,MotorDyn.D_theta,MotorDyn.K_theta,dq_init,q_init
  Product2 : Product  Multiplication=Matrix(*)  RndMeth=Zero
  Product4 : Product  Multiplication=Matrix(*)  RndMeth=Zero
  Product6 : Product  Inputs=/  Multiplication=Matrix(*)  RndMeth=Zero
  Product7 : Product  Multiplication=Matrix(*)  RndMeth=Zero
  Sum1 : Sum
  Sum2 : Sum  Inputs=-+|
  Sum3 : Sum  Inputs=-+|
  Sum5 : Sum  Inputs=--+
  output dtheta : Integrator  InitialConditionSource=external  InitialCondition=[zeros(Nb,1); dq_init]
  output theta : Integrator  InitialConditionSource=external  InitialCondition=[zeros(Nb,1); dq_init]
  tau_link : Outport
  theta : Outport  Port=2
  dtheta : Outport  Port=3
  wires:
  Bus Selector1/4 -> output dtheta/2  "<dq_init>"
  output dtheta/1 -> output theta/1, dtheta/1, Sum2/2  "dtheta"
  Product7/1 -> output dtheta/1  "ddtheta"
  Sum5/1 -> Product7/2
  Bus Selector1/1 -> Product6/1  "<B_theta>"
  Bus Selector1/3 -> Product4/1  "<K_theta>"
  tau_m/1 -> Sum5/3
  Bus Selector1/5 -> output theta/2  "<q_init>"
  Product6/1 -> Product7/1
  Sum2/1 -> Product2/2
  Bus Selector1/2 -> Product2/1  "<D_theta>"
  Product4/1 -> Sum1/2, Sum5/2
  Sum3/1 -> Product4/2
  output theta/1 -> theta/1, Sum3/2  "theta"
  dq/1 -> Sum2/1  "dq"
  q/1 -> Sum3/1  "q"
  Product2/1 -> Sum1/1, Sum5/1
  parameters/1 -> Bus Selector1/1
  Sum1/1 -> tau_link/1

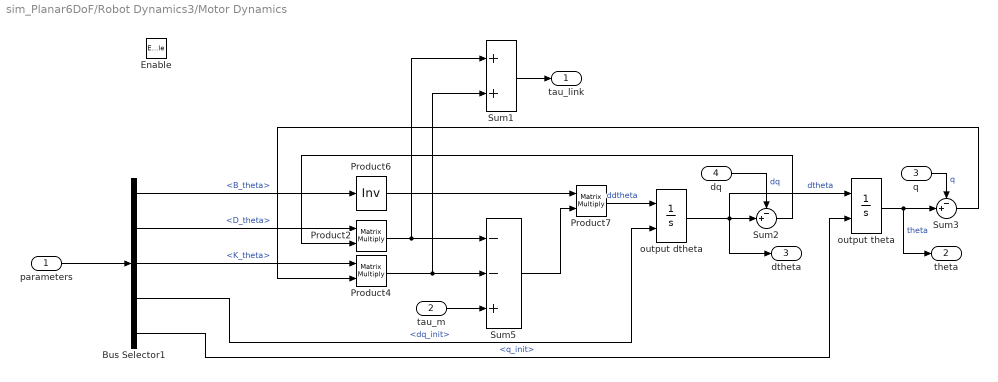
== system sim_Planar6DoF/Robot Dynamics3/Motor Dynamics ==
  parameters : Inport
  tau_m : Inport  Port=2
  q : Inport  Port=3
  dq : Inport  Port=4
  Enable : EnablePort
  Bus Selector1 : BusSelector  OutputSignals=MotorDyn.B_theta,MotorDyn.D_theta,MotorDyn.K_theta,dq_init,q_init
  Product2 : Product  Multiplication=Matrix(*)  RndMeth=Zero
  Product4 : Product  Multiplication=Matrix(*)  RndMeth=Zero
  Product6 : Product  Inputs=/  Multiplication=Matrix(*)  RndMeth=Zero
  Product7 : Product  Multiplication=Matrix(*)  RndMeth=Zero
  Sum1 : Sum
  Sum2 : Sum  Inputs=-+|
  Sum3 : Sum  Inputs=-+|
  Sum5 : Sum  Inputs=--+
  output dtheta : Integrator  InitialConditionSource=external  InitialCondition=[zeros(Nb,1); dq_init]
  output theta : Integrator  InitialConditionSource=external  InitialCondition=[zeros(Nb,1); dq_init]
  tau_link : Outport
  theta : Outport  Port=2
  dtheta : Outport  Port=3
  wires:
  Sum1/1 -> tau_link/1
  parameters/1 -> Bus Selector1/1
  Product2/1 -> Sum5/1, Sum1/1
  q/1 -> Sum3/1  "q"
  dq/1 -> Sum2/1  "dq"
  output theta/1 -> Sum3/2, theta/1  "theta"
  Sum3/1 -> Product4/2
  Product4/1 -> Sum5/2, Sum1/2
  Bus Selector1/2 -> Product2/1  "<D_theta>"
  Sum2/1 -> Product2/2
  Product6/1 -> Product7/1
  Bus Selector1/5 -> output theta/2  "<q_init>"
  tau_m/1 -> Sum5/3
  Bus Selector1/3 -> Product4/1  "<K_theta>"
  Bus Selector1/1 -> Product6/1  "<B_theta>"
  Sum5/1 -> Product7/2
  Product7/1 -> output dtheta/1  "ddtheta"
  output dtheta/1 -> Sum2/2, dtheta/1, output theta/1  "dtheta"
  Bus Selector1/4 -> output dtheta/2  "<dq_init>"

== system sim_Planar6DoF/Robust Controller/Storage Function ==
  M : Inport
  K : Inport  Port=2
  e : Inport  Port=3
  de : Inport  Port=4
  Add1 : Sum
  Gain : Gain  Gain=0.5
  Math Function : Math  Operator=transpose  SaturateOnIntegerOverflow=on
  Math Function1 : Math  Operator=transpose  SaturateOnIntegerOverflow=on
  Product{1..4} (4 alike) : Product  Multiplication=Matrix(*)  RndMeth=Zero
  V_kin : Scope
  V_pot : Scope
  V_total : Scope
  V : Outport
  wires:
  Product2/1 -> Gain/1
  Gain/1 -> Add1/1, V_kin/1
  Product4/1 -> Product2/1
  de/1 -> Product2/2, Math Function/1
  Math Function/1 -> Product4/1
  M/1 -> Product4/2
  K/1 -> Product3/2
  Math Function1/1 -> Product3/1
  e/1 -> Product1/2, Math Function1/1
  Product3/1 -> Product1/1
  Product1/1 -> Add1/2, V_pot/1
  Add1/1 -> V_total/1, V/1

== system sim_Planar6DoF/Trajectory Generator/Regulation Traj ==
  Enable : EnablePort
  dev_q : Subsystem  mask{amplitude_input=[-0.2, 10*pi/180*ones(1, 5)], t_wait=0.5, t_fw=0.01, t_hold=2, t_bw=0.01}
      mask prompts: amplitude_input "Amplitude"; t_wait "Time for waiting"; t_fw "Time for forward trajectory"; t_hold "Time for holding"; t_bw "Time for backward trajectory"
  q_dev : Outport  InitialOutput=zeros(6,1)
  dq_des : Outport  Port=2  InitialOutput=zeros(6,1)
  ddq_des : Outport  Port=3  InitialOutput=zeros(6,1)
  wires:
  dev_q/1(q_dev) -> q_dev/1
  dev_q/2(dq_des) -> dq_des/1
  dev_q/3(ddq_des) -> ddq_des/1

== system sim_Planar6DoF/Trajectory Generator/Tracking Traj ==
  Enable : EnablePort
  Constant12 : Constant  Value=q0_offset  SampleTime=-1
  Sum : Sum  Inputs=++|
  dev_q : Subsystem  mask{amplitude_input=[-0.2, pi/180*[-10, 10, -10, -5, -5]], f_input=1}
      mask prompts: amplitude_input "Amplitude"; f_input "Frequency [Hz]"
  q_dev : Outport  InitialOutput=zeros(6,1)
  dq_des : Outport  Port=2  InitialOutput=zeros(6,1)
  ddq_des : Outport  Port=3  InitialOutput=zeros(6,1)
  wires:
  Constant12/1 -> Sum/1
  Sum/1 -> q_dev/1
  dev_q/1(q_dev) -> Sum/2
  dev_q/2(dq_des) -> dq_des/1
  dev_q/3(ddq_des) -> ddq_des/1

== system sim_Planar6DoF/Trajectory Generator/Regulation Traj/dev_q ==
  Constant2 : Constant  Value=zeros(6,1)
  Discrete PT2 : Subsystem  mask{T=10*Ts, D=1}
  Mux : Mux  Inputs=6
  dev_q1 : Subsystem
  dev_q2 : Subsystem
  dev_q3 : Subsystem
  dev_q4 : Subsystem
  dev_q5 : Subsystem
  dev_q6 : Subsystem
  q_dev : Outport  InitialOutput=zeros(6,1)
  dq_des : Outport  Port=2  InitialOutput=zeros(6,1)
  ddq_des : Outport  Port=3  InitialOutput=zeros(6,1)
  wires:
  dev_q1/1(q_d) -> Mux/1
  dev_q3/1(q_d) -> Mux/3
  Mux/1 -> Discrete PT2/1(q_d)
  dev_q5/1(q_d) -> Mux/5
  dev_q4/1(q_d) -> Mux/4
  dev_q2/1(q_d) -> Mux/2
  Constant2/1 -> ddq_des/1, dq_des/1
  dev_q6/1(q_d) -> Mux/6
  Discrete PT2/1(q_filt) -> q_dev/1

== system sim_Planar6DoF/Trajectory Generator/Tracking Traj/dev_q ==
  Mux1 : Mux  Inputs=6
  Mux2 : Mux  Inputs=6
  Mux3 : Mux  Inputs=6
  dev_q1 : Subsystem
  dev_q2 : Subsystem
  dev_q3 : Subsystem
  dev_q4 : Subsystem
  dev_q5 : Subsystem
  dev_q6 : Subsystem
  q_dev : Outport  InitialOutput=zeros(6,1)
  dq_des : Outport  Port=2  InitialOutput=zeros(6,1)
  ddq_des : Outport  Port=3  InitialOutput=zeros(6,1)
  wires:
  Mux1/1 -> q_dev/1
  dev_q5/3(ddy) -> Mux3/5
  dev_q4/2(dy) -> Mux2/4
  dev_q4/3(ddy) -> Mux3/4
  dev_q6/3(ddy) -> Mux3/6
  dev_q3/3(ddy) -> Mux3/3
  dev_q5/2(dy) -> Mux2/5
  dev_q2/2(dy) -> Mux2/2
  dev_q5/1(y) -> Mux1/5
  dev_q3/1(y) -> Mux1/3
  dev_q2/1(y) -> Mux1/2
  dev_q1/1(y) -> Mux1/1
  dev_q6/1(y) -> Mux1/6
  dev_q4/1(y) -> Mux1/4
  dev_q6/2(dy) -> Mux2/6
  dev_q2/3(ddy) -> Mux3/2
  dev_q1/3(ddy) -> Mux3/1
  dev_q1/2(dy) -> Mux2/1
  dev_q3/2(dy) -> Mux2/3
  Mux3/1 -> ddq_des/1
  Mux2/1 -> dq_des/1

== system sim_Planar6DoF/Trajectory Generator/Regulation Traj/dev_q/Discrete PT2 ==
  q_d : Inport
  Add : Sum  Inputs=+--
  Discrete-Time Integrator1 : DiscreteIntegrator  InitialConditionSetting=State (most efficient)  SampleTime=Ts  ICPrevOutput=DiscIntNeverNeededParam  ICPrevScaledInput=DiscIntNeverNeededParam
  Discrete-Time Integrator2 : DiscreteIntegrator  InitialConditionSetting=State (most efficient)  SampleTime=Ts  ICPrevOutput=DiscIntNeverNeededParam  ICPrevScaledInput=DiscIntNeverNeededParam
  Gain : Gain  Gain=1/T^2
  Gain1 : Gain  Gain=2*D/T
  Gain2 : Gain  Gain=1/T^2
  q_filt : Outport
  wires:
  Gain1/1 -> Add/2
  Discrete-Time Integrator1/1 -> Gain1/1, Discrete-Time Integrator2/1  "dq"
  q_d/1 -> Gain/1
  Discrete-Time Integrator2/1 -> Gain2/1, q_filt/1  "q"
  Add/1 -> Discrete-Time Integrator1/1  "ddq"
  Gain/1 -> Add/1
  Gain2/1 -> Add/3

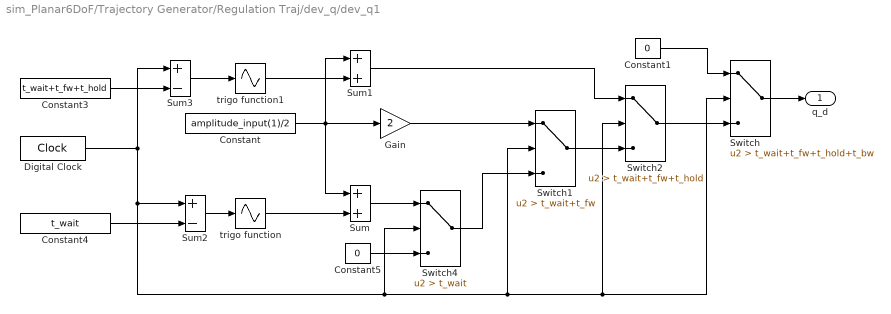
== system sim_Planar6DoF/Trajectory Generator/Regulation Traj/dev_q/dev_q1 ==
  Constant : Constant  Value=amplitude_input(1)/2
  Constant1 : Constant  Value=0
  Constant3 : Constant  Value=t_wait+t_fw+t_hold
  Constant4 : Constant  Value=t_wait
  Constant5 : Constant  Value=0
  Digital Clock : DigitalClock  SampleTime=Ts
  Gain : Gain  Gain=2
  Sum : Sum
  Sum1 : Sum
  Sum2 : Sum  Inputs=+-
  Sum3 : Sum  Inputs=+-
  Switch : Switch  Criteria=u2 > Threshold  Threshold=t_wait+t_fw+t_hold+t_bw
  Switch1 : Switch  Criteria=u2 > Threshold  Threshold=t_wait+t_fw
  Switch2 : Switch  Criteria=u2 > Threshold  Threshold=t_wait+t_fw+t_hold
  Switch4 : Switch  Criteria=u2 > Threshold  Threshold=t_wait
  trigo function : Sin  TimeSource=Use external signal  Amplitude=-amplitude_input(1)/2  Frequency=2*pi/(2*t_fw)  Phase=pi/2  SampleTime=0
  trigo function1 : Sin  TimeSource=Use external signal  Amplitude=-amplitude_input(1)/2  Frequency=2*pi/(2*t_bw)  Phase=-pi/2  SampleTime=0
  q_d : Outport
  wires:
  Switch/1 -> q_d/1
  Sum/1 -> Switch4/1
  Constant1/1 -> Switch/1
  trigo function/1 -> Sum/2
  Constant/1 -> Sum/1, Sum1/1, Gain/1
  Switch1/1 -> Switch2/3
  Gain/1 -> Switch1/1
  Switch2/1 -> Switch/3
  Sum1/1 -> Switch2/1
  Sum3/1 -> trigo function1/1
  Constant3/1 -> Sum3/2
  trigo function1/1 -> Sum1/2
  Digital Clock/1 -> Switch4/2, Switch1/2, Switch2/2, Switch/2, Sum2/1, Sum3/1
  Constant4/1 -> Sum2/2
  Sum2/1 -> trigo function/1
  Switch4/1 -> Switch1/3
  Constant5/1 -> Switch4/3

== system sim_Planar6DoF/Trajectory Generator/Regulation Traj/dev_q/dev_q2 ==
  Constant : Constant  Value=amplitude_input(2)/2
  Constant1 : Constant  Value=0
  Constant3 : Constant  Value=t_wait+t_fw+t_hold
  Constant4 : Constant  Value=t_wait
  Constant5 : Constant  Value=0
  Digital Clock : DigitalClock  SampleTime=Ts
  Gain : Gain  Gain=2
  Sum : Sum
  Sum1 : Sum
  Sum2 : Sum  Inputs=+-
  Sum3 : Sum  Inputs=+-
  Switch : Switch  Criteria=u2 > Threshold  Threshold=t_wait+t_fw+t_hold+t_bw
  Switch1 : Switch  Criteria=u2 > Threshold  Threshold=t_wait+t_fw
  Switch2 : Switch  Criteria=u2 > Threshold  Threshold=t_wait+t_fw+t_hold
  Switch4 : Switch  Criteria=u2 > Threshold  Threshold=t_wait
  trigo function : Sin  TimeSource=Use external signal  Amplitude=-amplitude_input(2)/2  Frequency=2*pi/(2*t_fw)  Phase=pi/2  SampleTime=0
  trigo function1 : Sin  TimeSource=Use external signal  Amplitude=-amplitude_input(2)/2  Frequency=2*pi/(2*t_bw)  Phase=-pi/2  SampleTime=0
  q_d : Outport
  wires:
  Constant5/1 -> Switch4/3
  Switch4/1 -> Switch1/3
  Sum2/1 -> trigo function/1
  Constant4/1 -> Sum2/2
  Digital Clock/1 -> Sum3/1, Sum2/1, Switch/2, Switch2/2, Switch1/2, Switch4/2
  trigo function1/1 -> Sum1/2
  Constant3/1 -> Sum3/2
  Sum3/1 -> trigo function1/1
  Sum1/1 -> Switch2/1
  Switch2/1 -> Switch/3
  Gain/1 -> Switch1/1
  Switch1/1 -> Switch2/3
  Constant/1 -> Gain/1, Sum1/1, Sum/1
  trigo function/1 -> Sum/2
  Constant1/1 -> Switch/1
  Sum/1 -> Switch4/1
  Switch/1 -> q_d/1

== system sim_Planar6DoF/Trajectory Generator/Regulation Traj/dev_q/dev_q3 ==
  Constant : Constant  Value=amplitude_input(3)/2
  Constant1 : Constant  Value=0
  Constant3 : Constant  Value=t_wait+t_fw+t_hold
  Constant4 : Constant  Value=t_wait
  Constant5 : Constant  Value=0
  Digital Clock : DigitalClock  SampleTime=Ts
  Gain : Gain  Gain=2
  Sum : Sum
  Sum1 : Sum
  Sum2 : Sum  Inputs=+-
  Sum3 : Sum  Inputs=+-
  Switch : Switch  Criteria=u2 > Threshold  Threshold=t_wait+t_fw+t_hold+t_bw
  Switch1 : Switch  Criteria=u2 > Threshold  Threshold=t_wait+t_fw
  Switch2 : Switch  Criteria=u2 > Threshold  Threshold=t_wait+t_fw+t_hold
  Switch4 : Switch  Criteria=u2 > Threshold  Threshold=t_wait
  trigo function : Sin  TimeSource=Use external signal  Amplitude=-amplitude_input(3)/2  Frequency=2*pi/(2*t_fw)  Phase=pi/2  SampleTime=0
  trigo function1 : Sin  TimeSource=Use external signal  Amplitude=-amplitude_input(3)/2  Frequency=2*pi/(2*t_bw)  Phase=-pi/2  SampleTime=0
  q_d : Outport
  wires:
  Switch/1 -> q_d/1
  Sum/1 -> Switch4/1
  Constant1/1 -> Switch/1
  trigo function/1 -> Sum/2
  Constant/1 -> Sum/1, Sum1/1, Gain/1
  Switch1/1 -> Switch2/3
  Gain/1 -> Switch1/1
  Switch2/1 -> Switch/3
  Sum1/1 -> Switch2/1
  Sum3/1 -> trigo function1/1
  Constant3/1 -> Sum3/2
  trigo function1/1 -> Sum1/2
  Digital Clock/1 -> Switch4/2, Switch1/2, Switch2/2, Switch/2, Sum2/1, Sum3/1
  Constant4/1 -> Sum2/2
  Sum2/1 -> trigo function/1
  Switch4/1 -> Switch1/3
  Constant5/1 -> Switch4/3

== system sim_Planar6DoF/Trajectory Generator/Regulation Traj/dev_q/dev_q4 ==
  Constant : Constant  Value=amplitude_input(4)/2
  Constant1 : Constant  Value=0
  Constant3 : Constant  Value=t_wait+t_fw+t_hold
  Constant4 : Constant  Value=t_wait
  Constant5 : Constant  Value=0
  Digital Clock : DigitalClock  SampleTime=Ts
  Gain : Gain  Gain=2
  Sum : Sum
  Sum1 : Sum
  Sum2 : Sum  Inputs=+-
  Sum3 : Sum  Inputs=+-
  Switch : Switch  Criteria=u2 > Threshold  Threshold=t_wait+t_fw+t_hold+t_bw
  Switch1 : Switch  Criteria=u2 > Threshold  Threshold=t_wait+t_fw
  Switch2 : Switch  Criteria=u2 > Threshold  Threshold=t_wait+t_fw+t_hold
  Switch4 : Switch  Criteria=u2 > Threshold  Threshold=t_wait
  trigo function : Sin  TimeSource=Use external signal  Amplitude=-amplitude_input(4)/2  Frequency=2*pi/(2*t_fw)  Phase=pi/2  SampleTime=0
  trigo function1 : Sin  TimeSource=Use external signal  Amplitude=-amplitude_input(4)/2  Frequency=2*pi/(2*t_bw)  Phase=-pi/2  SampleTime=0
  q_d : Outport
  wires:
  Constant5/1 -> Switch4/3
  Switch4/1 -> Switch1/3
  Sum2/1 -> trigo function/1
  Constant4/1 -> Sum2/2
  Digital Clock/1 -> Sum3/1, Sum2/1, Switch/2, Switch2/2, Switch1/2, Switch4/2
  trigo function1/1 -> Sum1/2
  Constant3/1 -> Sum3/2
  Sum3/1 -> trigo function1/1
  Sum1/1 -> Switch2/1
  Switch2/1 -> Switch/3
  Gain/1 -> Switch1/1
  Switch1/1 -> Switch2/3
  Constant/1 -> Gain/1, Sum1/1, Sum/1
  trigo function/1 -> Sum/2
  Constant1/1 -> Switch/1
  Sum/1 -> Switch4/1
  Switch/1 -> q_d/1

== system sim_Planar6DoF/Trajectory Generator/Regulation Traj/dev_q/dev_q5 ==
  Constant : Constant  Value=amplitude_input(5)/2
  Constant1 : Constant  Value=0
  Constant3 : Constant  Value=t_wait+t_fw+t_hold
  Constant4 : Constant  Value=t_wait
  Constant5 : Constant  Value=0
  Digital Clock : DigitalClock  SampleTime=Ts
  Gain : Gain  Gain=2
  Sum : Sum
  Sum1 : Sum
  Sum2 : Sum  Inputs=+-
  Sum3 : Sum  Inputs=+-
  Switch : Switch  Criteria=u2 > Threshold  Threshold=t_wait+t_fw+t_hold+t_bw
  Switch1 : Switch  Criteria=u2 > Threshold  Threshold=t_wait+t_fw
  Switch2 : Switch  Criteria=u2 > Threshold  Threshold=t_wait+t_fw+t_hold
  Switch4 : Switch  Criteria=u2 > Threshold  Threshold=t_wait
  trigo function : Sin  TimeSource=Use external signal  Amplitude=-amplitude_input(5)/2  Frequency=2*pi/(2*t_fw)  Phase=pi/2  SampleTime=0
  trigo function1 : Sin  TimeSource=Use external signal  Amplitude=-amplitude_input(5)/2  Frequency=2*pi/(2*t_bw)  Phase=-pi/2  SampleTime=0
  q_d : Outport
  wires:
  Switch/1 -> q_d/1
  Sum/1 -> Switch4/1
  Constant1/1 -> Switch/1
  trigo function/1 -> Sum/2
  Constant/1 -> Sum/1, Sum1/1, Gain/1
  Switch1/1 -> Switch2/3
  Gain/1 -> Switch1/1
  Switch2/1 -> Switch/3
  Sum1/1 -> Switch2/1
  Sum3/1 -> trigo function1/1
  Constant3/1 -> Sum3/2
  trigo function1/1 -> Sum1/2
  Digital Clock/1 -> Switch4/2, Switch1/2, Switch2/2, Switch/2, Sum2/1, Sum3/1
  Constant4/1 -> Sum2/2
  Sum2/1 -> trigo function/1
  Switch4/1 -> Switch1/3
  Constant5/1 -> Switch4/3

== system sim_Planar6DoF/Trajectory Generator/Regulation Traj/dev_q/dev_q6 ==
  Constant : Constant  Value=amplitude_input(6)/2
  Constant1 : Constant  Value=0
  Constant3 : Constant  Value=t_wait+t_fw+t_hold
  Constant4 : Constant  Value=t_wait
  Constant5 : Constant  Value=0
  Digital Clock : DigitalClock  SampleTime=Ts
  Gain : Gain  Gain=2
  Sum : Sum
  Sum1 : Sum
  Sum2 : Sum  Inputs=+-
  Sum3 : Sum  Inputs=+-
  Switch : Switch  Criteria=u2 > Threshold  Threshold=t_wait+t_fw+t_hold+t_bw
  Switch1 : Switch  Criteria=u2 > Threshold  Threshold=t_wait+t_fw
  Switch2 : Switch  Criteria=u2 > Threshold  Threshold=t_wait+t_fw+t_hold
  Switch4 : Switch  Criteria=u2 > Threshold  Threshold=t_wait
  trigo function : Sin  TimeSource=Use external signal  Amplitude=-amplitude_input(6)/2  Frequency=2*pi/(2*t_fw)  Phase=pi/2  SampleTime=0
  trigo function1 : Sin  TimeSource=Use external signal  Amplitude=-amplitude_input(6)/2  Frequency=2*pi/(2*t_bw)  Phase=-pi/2  SampleTime=0
  q_d : Outport
  wires:
  Constant5/1 -> Switch4/3
  Switch4/1 -> Switch1/3
  Sum2/1 -> trigo function/1
  Constant4/1 -> Sum2/2
  Digital Clock/1 -> Sum3/1, Sum2/1, Switch/2, Switch2/2, Switch1/2, Switch4/2
  trigo function1/1 -> Sum1/2
  Constant3/1 -> Sum3/2
  Sum3/1 -> trigo function1/1
  Sum1/1 -> Switch2/1
  Switch2/1 -> Switch/3
  Gain/1 -> Switch1/1
  Switch1/1 -> Switch2/3
  Constant/1 -> Gain/1, Sum1/1, Sum/1
  trigo function/1 -> Sum/2
  Constant1/1 -> Switch/1
  Sum/1 -> Switch4/1
  Switch/1 -> q_d/1
